simulink model "txt_gen"  (R2024b)
settings: Solver=VariableStepAuto  StartTime=0.0  StopTime=20  RelTol=1e-3
values from neighbouring files (symbols this model uses):
  f_au = 48e3    (= 48000)    [duc_data_gen.m]
  fs = 120e6    (= 120000000)    [duc_data_analyse.m]    (also in duc_data_gen.m)
  length_score_music = length(vec_score_music)    [audio_gen.m]
  phInc_base_1 = ceil((f_base_1*2^Nnco*up_L)/fs)    [duc_data_gen.m]
  phInc_base_2 = ceil((f_base_2*2^Nnco*up_L)/fs)    [duc_data_gen.m]
  sample_times_one_note = fix(time_one_note*f_au)    [audio_gen.m]
  up_L = fs/f_au    (= 2500)    [duc_data_gen.m]
libraries: hdlsllib x4, dsphdlsigops2 x3, simulink x1
settings Model: Creator=31651  LastModifiedBy=31651

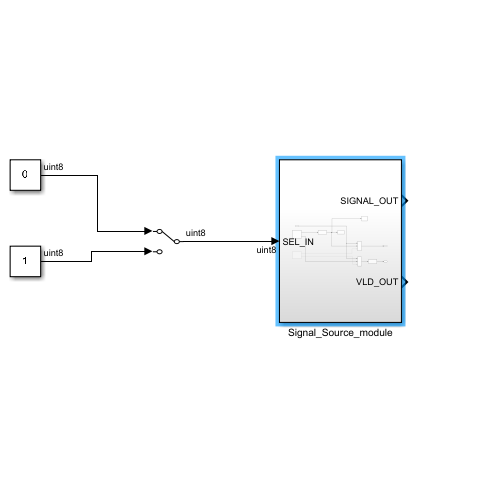
[thumbnail: Simulink's stored preview of the top-level diagram]
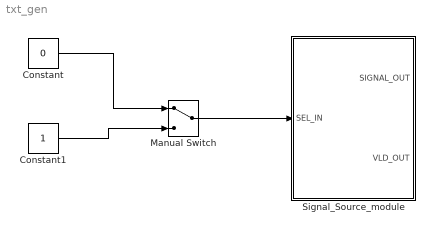
== system txt_gen ==
  Constant : Constant  Value=0  OutDataTypeStr=uint8
  Constant1 : Constant  OutDataTypeStr=uint8
  Manual Switch : ManualSwitch
  Signal_Source_module : Subsystem
  wires:
  Constant/1 -> Manual Switch/1
  Manual Switch/1 -> Signal_Source_module/1(SEL_IN)
  Constant1/1 -> Manual Switch/2

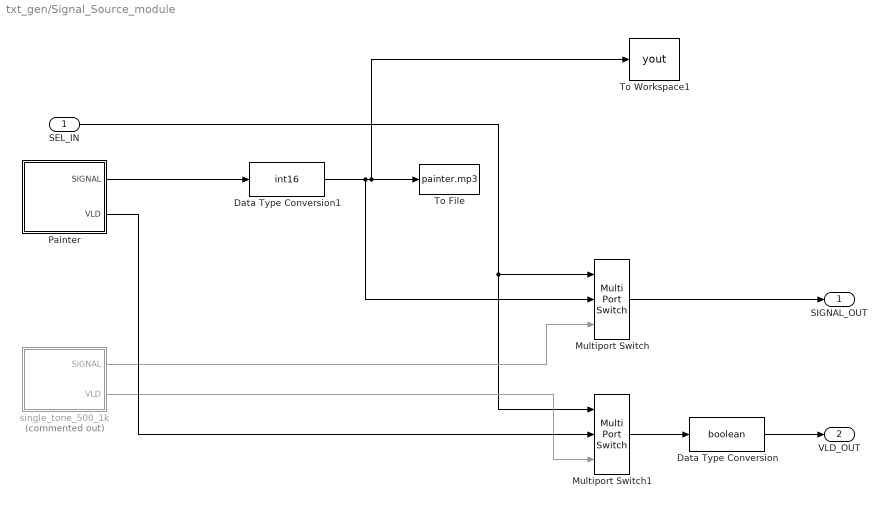
== system txt_gen/Signal_Source_module ==
  SEL_IN : Inport  OutDataTypeStr=uint8
  Data Type Conversion : DataTypeConversion  OutDataTypeStr=boolean  SaturateOnIntegerOverflow=off  RndMeth=Floor
  Data Type Conversion1 : DataTypeConversion  OutDataTypeStr=int16  ConvertRealWorld=Stored Integer (SI)  SaturateOnIntegerOverflow=off  RndMeth=Floor
  Multiport Switch : MultiPortSwitch  DataPortOrder=Zero-based contiguous  Inputs=2  zeroidx=on  OutDataTypeStr=fixdt(1,16,15)  SaturateOnIntegerOverflow=off  InputSameDT=off
  Multiport Switch1 : MultiPortSwitch  DataPortOrder=Zero-based contiguous  Inputs=2  zeroidx=on  OutDataTypeStr=fixdt(1,16,15)  SaturateOnIntegerOverflow=off  InputSameDT=off
  Painter : Subsystem
  To File : ToFile  Filename=painter.mp3  SaveFormat=Timeseries
  To Workspace1 : ToWorkspace  VariableName=yout  SampleTime=-1
      settings: Save2DSignal=2-D array (concatenate along first dimension)
  single_tone_500_1k : Subsystem  Commented=on
  SIGNAL_OUT : Outport
  VLD_OUT : Outport  Port=2  OutDataTypeStr=boolean
  wires:
  Multiport Switch/1 -> SIGNAL_OUT/1
  Multiport Switch1/1 -> Data Type Conversion/1
  SEL_IN/1 -> Multiport Switch1/1, Multiport Switch/1
  Data Type Conversion/1 -> VLD_OUT/1
  single_tone_500_1k/1(SIGNAL) -> Multiport Switch/3
  single_tone_500_1k/2(VLD) -> Multiport Switch1/3
  Painter/1(SIGNAL) -> Data Type Conversion1/1
  Painter/2(VLD) -> Multiport Switch1/2
  Data Type Conversion1/1 -> To Workspace1/1, To File/1, Multiport Switch/2

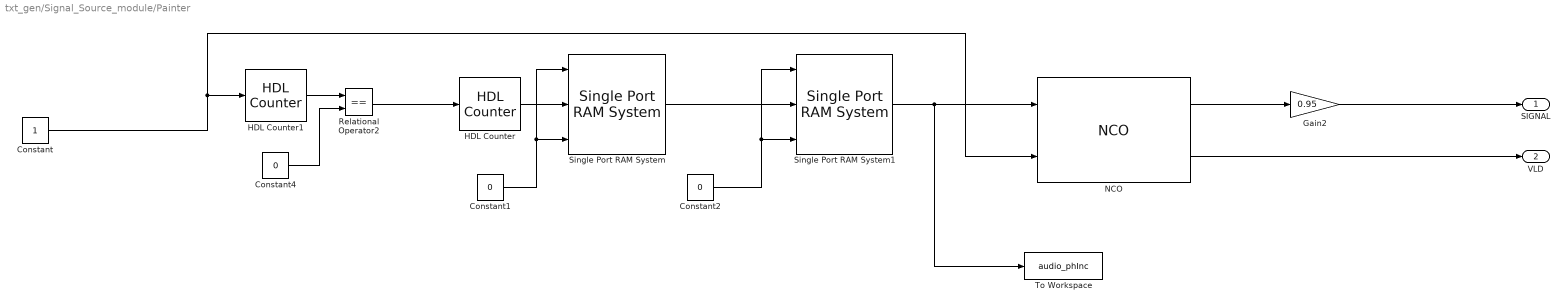
== system txt_gen/Signal_Source_module/Painter ==
  Constant : Constant  OutDataTypeStr=boolean  SampleTime=1/f_au
  Constant1 : Constant  Value=0  OutDataTypeStr=uint8  SampleTime=1/f_au
  Constant2 : Constant  Value=0  OutDataTypeStr=uint32  SampleTime=1/f_au
  Constant4 : Constant  Value=0  OutDataTypeStr=uint16  SampleTime=1/f_au
  Gain2 : Gain  Gain=0.95  OutDataTypeStr=fixdt(1,16,15)
  HDL Counter : hdlsllib/Sources/HDL Counter  CountType=Count limited  CountInit=0  CountStep=1  CountMax=length_score_music-1  CountFromType=Initial value  CountFrom=0  CountResetPort=off  CountLoadPort=off  CountEnbPort=on  CountDirPort=off  CountHitOutputPort=off  CountDataType=Unsigned  CountWordLen=8  CountFracLen=0  CountSampTime=1/f_au
  HDL Counter1 : hdlsllib/Sources/HDL Counter  CountType=Count limited  CountInit=0  CountStep=1  CountMax=sample_times_one_note-1  CountFromType=Initial value  CountFrom=0  CountResetPort=off  CountLoadPort=off  CountEnbPort=on  CountDirPort=off  CountHitOutputPort=off  CountDataType=Unsigned  CountWordLen=16  CountFracLen=0  CountSampTime=1/f_au
  NCO : dsphdlsigops2/NCO  PhaseIncrementSource=Input port  PhaseIncrement=100  PhaseOffsetSource=Property  PhaseOffset=0  DitherSource=Property  NumDitherBits=ditherBits  SamplesPerFrame=1  LUTCompress=on  ResetAction=off  Waveform=Sine  PhasePort=off  SimulateUsing=Code generation  AccumulatorWL=Nnco  PhaseQuantization=on  NumQuantizerAccumulatorBits=Q  OutputDataType=Binary point scaling  OutputWL=16  OutputFL=15
  Relational Operator2 : RelationalOperator  Operator===  OutDataTypeStr=boolean  RndMeth=Simplest  InputSameDT=off
  Single Port RAM System : hdlsllib/HDL RAMs/Single Port RAM System  RAMType=Single port  AsyncRead=off  WriteOutputValue=New data  RAMInitialValue=vec_score_music  allowBusInputs=off  WritesHaveOutput=on  NumReads=0  NumWrites=1  SimulateUsing=Code generation  ModelRAMDelay=on
  Single Port RAM System1 : hdlsllib/HDL RAMs/Single Port RAM System  RAMType=Single port  AsyncRead=on  WriteOutputValue=New data  RAMInitialValue=vec_freq_music_phinc  allowBusInputs=off  WritesHaveOutput=on  NumReads=0  NumWrites=1  SimulateUsing=Code generation  ModelRAMDelay=on
  To Workspace : ToWorkspace  VariableName=audio_phInc  SaveFormat=Timeseries  SampleTime=-1
  SIGNAL : Outport
  VLD : Outport  Port=2
  wires:
  Constant/1 -> NCO/2, HDL Counter1/1
  Single Port RAM System1/1 -> To Workspace/1, NCO/1
  NCO/2 -> VLD/1
  HDL Counter1/1 -> Relational Operator2/1
  Constant2/1 -> Single Port RAM System1/3, Single Port RAM System1/1
  Constant1/1 -> Single Port RAM System/1, Single Port RAM System/3
  NCO/1 -> Gain2/1
  Single Port RAM System/1 -> Single Port RAM System1/2
  HDL Counter/1 -> Single Port RAM System/2
  Relational Operator2/1 -> HDL Counter/1
  Constant4/1 -> Relational Operator2/2
  Gain2/1 -> SIGNAL/1

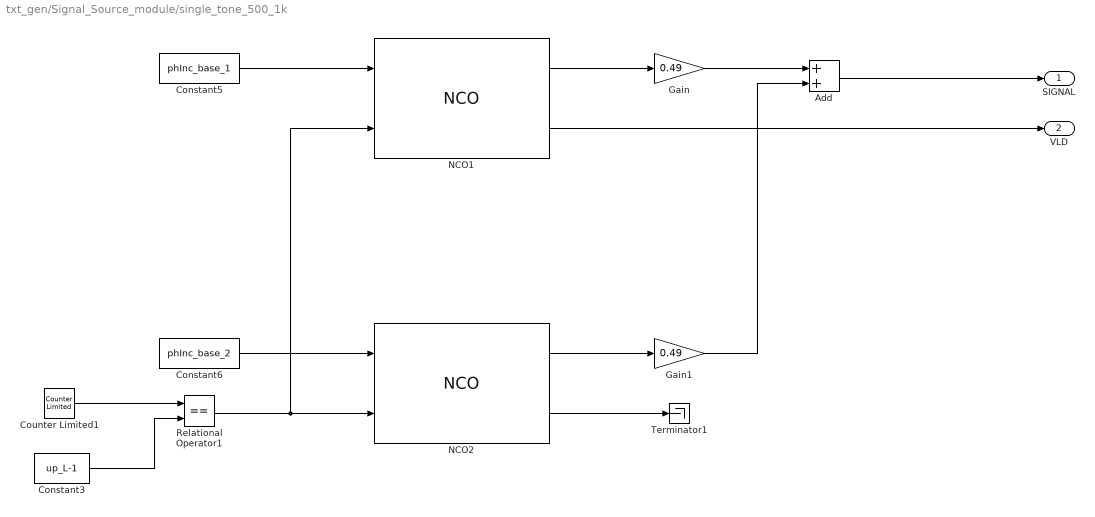
== system txt_gen/Signal_Source_module/single_tone_500_1k ==
  Add : Sum
  Constant3 : Constant  Value=up_L-1  OutDataTypeStr=uint16  SampleTime=1/fs
  Constant5 : Constant  Value=phInc_base_1  OutDataTypeStr=uint32  SampleTime=1/fs
  Constant6 : Constant  Value=phInc_base_2  OutDataTypeStr=uint32  SampleTime=1/fs
  Counter Limited1 : simulink/Sources/Counter Limited  uplimit=up_L-1  tsamp=1/fs
  Gain : Gain  Gain=0.49  OutDataTypeStr=Inherit: Same as input
  Gain1 : Gain  Gain=0.49  OutDataTypeStr=Inherit: Same as input
  NCO1 : dsphdlsigops2/NCO  PhaseIncrementSource=Input port  PhaseIncrement=100  PhaseOffsetSource=Property  PhaseOffset=0  DitherSource=Property  NumDitherBits=ditherBits  SamplesPerFrame=1  LUTCompress=off  ResetAction=off  Waveform=Sine  PhasePort=off  SimulateUsing=Code generation  AccumulatorWL=Nnco  PhaseQuantization=on  NumQuantizerAccumulatorBits=Q  OutputDataType=Binary point scaling  OutputWL=16  OutputFL=15
  NCO2 : dsphdlsigops2/NCO  PhaseIncrementSource=Input port  PhaseIncrement=100  PhaseOffsetSource=Property  PhaseOffset=0  DitherSource=Property  NumDitherBits=ditherBits  SamplesPerFrame=1  LUTCompress=off  ResetAction=off  Waveform=Sine  PhasePort=off  SimulateUsing=Code generation  AccumulatorWL=Nnco  PhaseQuantization=on  NumQuantizerAccumulatorBits=Q  OutputDataType=Binary point scaling  OutputWL=16  OutputFL=15
  Relational Operator1 : RelationalOperator  Operator===  OutDataTypeStr=boolean  RndMeth=Simplest  InputSameDT=off
  Terminator1 : Terminator
  SIGNAL : Outport
  VLD : Outport  Port=2
  wires:
  NCO2/1 -> Gain1/1
  Gain1/1 -> Add/2
  NCO1/1 -> Gain/1
  Constant3/1 -> Relational Operator1/2
  Counter Limited1/1 -> Relational Operator1/1
  Constant5/1 -> NCO1/1
  NCO2/2 -> Terminator1/1
  Constant6/1 -> NCO2/1
  Gain/1 -> Add/1
  Relational Operator1/1 -> NCO1/2, NCO2/2
  Add/1 -> SIGNAL/1
  NCO1/2 -> VLD/1
